simulink model "DTC_"  (R2023b)
settings: Solver=ode23tb  StartTime=0.0  StopTime=0.4  RelTol=1e-4
libraries: spsDCVoltageSourceLib x1, spsGroundLib x1, spsPermanentMagnetSynchronousMachineLib x1, spsThreePhaseVIMeasurementLib x1, spsUniversalBridgeLib x1, sps_lib x1
settings Model: Creator=rainy  LastModifiedBy=rainy
settings DebuggingCC: IgnoredZcDiagnostic=none

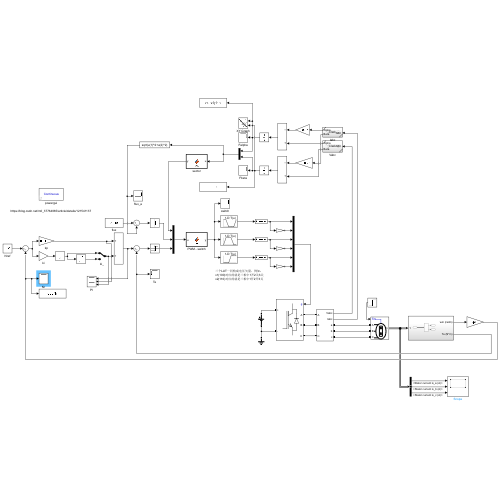
[thumbnail: Simulink's stored preview of the top-level diagram]
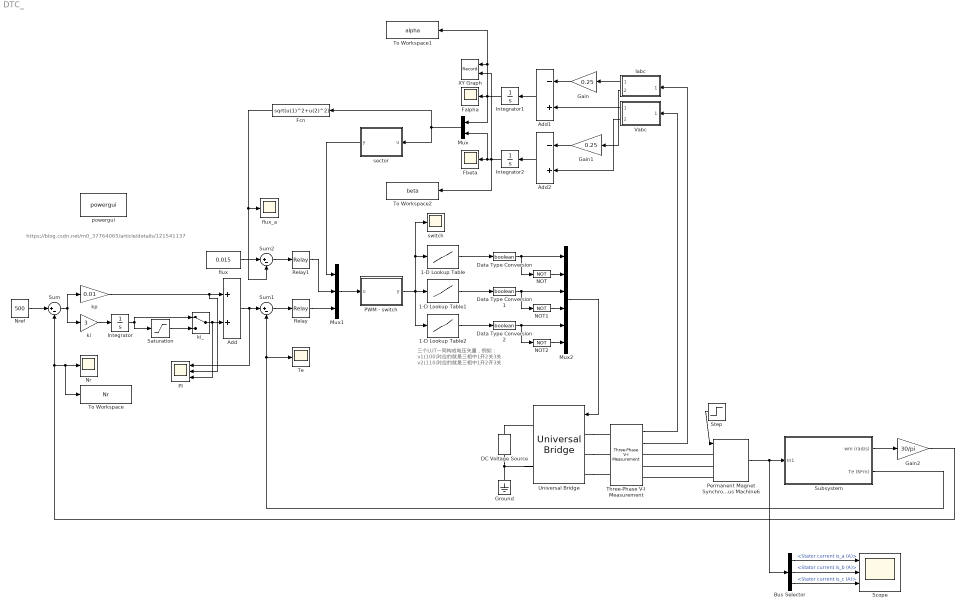
== system DTC_ ==
  note: 三个LUT一同构成电压矢量，例如：
      | v1(100)对应的就是三相中1开2关3关
      | v2(110)对应的就是三相中1开2开3关
  note: https://blog.csdn.net/m0_37764065/article/details/121541137
  1-D Lookup Table : Lookup_n-D  NumberOfTableDimensions=1  BreakpointsForDimension1=[1 2 3 4 5 6]  Table=[1 1 0 0 0 1]  InternalRulePriority=Speed  RndMeth=Simplest
  1-D Lookup Table1 : Lookup_n-D  NumberOfTableDimensions=1  BreakpointsForDimension1=[1 2 3 4 5 6]  Table=[0 1 1 1 0 0]  InternalRulePriority=Speed  RndMeth=Simplest
  1-D Lookup Table2 : Lookup_n-D  NumberOfTableDimensions=1  BreakpointsForDimension1=[1 2 3 4 5 6]  Table=[0 0 0 1 1 1]  InternalRulePriority=Speed  RndMeth=Simplest
  Add : Sum
  Add1 : Sum  Inputs=-+
  Add2 : Sum  Inputs=-+
  Bus Selector : BusSelector  OutputSignals=Stator current is_a (A),Stator current is_b (A),Stator current is_c (A)
  DC Voltage Source : spsDCVoltageSourceLib/DC Voltage Source  Amplitude=24  Measurements=Voltage
  Data Type Conversion : DataTypeConversion  OutDataTypeStr=boolean  SaturateOnIntegerOverflow=off  RndMeth=Floor
  Data Type Conversion1 : DataTypeConversion  OutDataTypeStr=boolean  SaturateOnIntegerOverflow=off  RndMeth=Floor
  Data Type Conversion2 : DataTypeConversion  OutDataTypeStr=boolean  SaturateOnIntegerOverflow=off  RndMeth=Floor
  Falpha : Scope
  Fbeta : Scope
  Fcn : Fcn  Expr=sqrt(u(1)^2+u(2)^2)
  Gain : Gain  Gain=0.25
  Gain1 : Gain  Gain=0.25
  Gain2 : Gain  Gain=30/pi
  Ground : spsGroundLib/Ground  LConnTagsString=a
  Iabc : Subsystem  ReferencedSubsystem=Clark
  Integrator : Integrator
  Integrator1 : Integrator
  Integrator2 : Integrator
  Mux : Mux  Inputs=2
  Mux1 : Mux  Inputs=3
  Mux2 : Mux  Inputs=6
  NOT : Logic  Operator=NOT  IconShape=distinctive  AllPortsSameDT=off  OutDataTypeStr=boolean
  NOT1 : Logic  Operator=NOT  IconShape=distinctive  AllPortsSameDT=off  OutDataTypeStr=boolean
  NOT2 : Logic  Operator=NOT  IconShape=distinctive  AllPortsSameDT=off  OutDataTypeStr=boolean
  Nr : Scope
  Nref : Constant  Value=500
  PI : Scope  NumInputPorts=3
  PWM - switch : MATLAB Function  TreatAsAtomicUnit=on
  Permanent Magnet Synchronous Machine6 : spsPermanentMagnetSynchronousMachineLib/Permanent Magnet Synchronous Machine  NbPhases=3  FluxDistribution=Sinusoidal  RotorType=Round  MechanicalLoad=Torque Tm  PresetModel=No  ShowDetailedParameters=on  MeasurementBus=off  Resistance=0.25  Inductance=8.5e-3  dqInductances=[8.5e-3,8.5e-3]  La=0.0005  MachineConstant=Flux linkage established by magnets (V.s)  Flux=0.01325  VoltageCst=9.6131  TorqueCst=0.0795  Flat=120  Mechanical=[0.00003 0 4 0]  PolePairs=4  InitialConditions=[0,0, 0,0]  InitialConditions5ph=[0 0 0 0 0 0]  RefAngle=Aligned with phase A axis (original Park)  IterativeDiscreteModel=Trapezoidal non iterative  TsBlock=-1  TsPowergui=0
  Relay : Relay  OnSwitchValue=0.01  OffSwitchValue=-0.01
  Relay1 : Relay  OnSwitchValue=0.002  OffSwitchValue=-0.002
  Saturation : Saturate  UpperLimit=10  LowerLimit=-10
  Scope : Scope  NumInputPorts=3
  Step : Step  Time=0.2  After=0.1  SampleTime=0
  Subsystem : Subsystem
  Sum : Sum  Inputs=|+-
  Sum1 : Sum  Inputs=|+-
  Sum2 : Sum  Inputs=|+-
  Te : Scope
  Three-Phase V-I Measurement : spsThreePhaseVIMeasurementLib/Three-Phase V-I Measurement  VoltageMeasurement=phase-to-ground  SetLabelV=off  LabelV=Vabc  Vpu=off  VpuLL=off  CurrentMeasurement=yes  SetLabelI=off  LabelI=Iabc  Ipu=off  Pbase=100e6  Vbase=500e3  OutputType=Complex  PhasorSimulation=off  PSBequivalent=0
  To Workspace : ToWorkspace  VariableName=Nr  SaveFormat=Timeseries  SampleTime=-1
  To Workspace1 : ToWorkspace  VariableName=alpha  SaveFormat=Timeseries  SampleTime=-1
  To Workspace2 : ToWorkspace  VariableName=beta  SaveFormat=Timeseries  SampleTime=-1
  Universal Bridge : spsUniversalBridgeLib/Universal Bridge  Arms=3  SnubberResistance=1e5  SnubberCapacitance=inf  Device=IGBT / Diodes  Ron=1e-3  Lon=0  ForwardVoltages="[  0  0  ]"  ForwardVoltage=0  GTOparameters=[ 10e-6 , 20e-6 ]  IGBTparameters=[ 1e-6 , 2e-6 ]  Measurements=None  Measurements_2=None  converterType=Rectifier
  Vabc : Subsystem  ReferencedSubsystem=Clark
  XY Graph : Record  FileSettingsInternal="{\"entries\":[{\"content\":{\"excelSettings\":{\"content\":{},\"type\":\"Streamout.ExcelSettings\"}},\"type\":\"Streamout.FileSettingStorage\",\"uuid\":\"\"}],\"packageUris\":[\"http:\\/\\/schema.mathworks.com\\/mf0\\/streamout_blocks\\/R2020a\"],\"version\":\"1.0\"}"  Layout=[1 1]  SignalsInternal="{\"entries\":[{\"content\":{\"signals\":[{\"content\":{\"blockPath\":[],\"dimensions\":[1],\"domain\":\"\",\"lineColor\":\"#22b573\",\"port\":1,\"sid\":[\"\"],\"signalID\":642,\"signalName\":\"Integrator1\"},\"type\":\"RecordBlkView.Signal\",\"uuid\":\"\"},{\"content\":{\"blockPath\":[],\"dimensions\":[1],\"domain\":\"\",\"lineColor\":\"#0072bd\",\"port\":2,\"sid\":[\"\"],\"signalID\":646,\"signalName\":\"Integrator2\"},\"type\":\"RecordBlkView.Signal\",\"uuid\":\"\"}]},\"type\":\"RecordBlkView.InputSignals\",\"uuid\":\"\"}],\"packageUris\":[\"http:\\/\\/schema.mathworks.com\\/mf0\\/streamout_blocks\\/R2020a\"],\"version\":\"1.0\"}"  VisualizationBindings="{\"xyplotplugin\":{\"info\":[{\"series\":[],\"subplotID\":1}]}}"  CompatibilityTag=XY  st=-1
  flux : Constant  Value=0.015
  flux_a : Scope
  ki : Gain  Gain=3
  ki_ : ManualSwitch
  kp : Gain  Gain=0.01
  powergui : sps_lib/powergui  Priority=1  SimulationMode=Continuous  SampleTime=50e-6  frequency=60  Iterations=50  frequencyindice=0  Pbase=100e6  ErrMax=1e-4  UnitsV=kV  UnitsW=MW  buscounter=0  FunctionMessages=off  echomessages=off  EnableUseOfTLC=off  CurrentSourceSwitches=off  DisableSnubberDevices=off  DisableRonSwitches=off  DisableVfSwitches=off  DisplayEquations=off  AutomaticDiscreteSolvers=off  SolverType=Tustin/Backward Euler (TBE)  Interpol=off  ExternalGateDelay=off  methode=off  Ts=100  x0status=blocks  SPID=on  SwTol=0  HookPort=off  NonlinearTolerance=1e-4  nMaxIteration=100  ContinueOnMaxIteration=off  RestoreLinks=warning  ResistiveCurrentMeasurement=off  Frange=[0:2:500]  Ylog=off  Xlog=on  ShowGrid=off  save=off  variable=ZData  structure=0  ZoomFFT=off  StartTime=0.0  cycles=1  DisplayStyle=1  fundamental=60  FreqAxis=off  MaxFrequency=1000  frequencyindicesteady=1  RmsSteady=1  display=off
  sector : MATLAB Function  TreatAsAtomicUnit=on
  switch : Scope
  wires:
  Sum/1 -> ki/1, kp/1
  ki/1 -> Integrator/1
  kp/1 -> PI/2, Add/1
  Add/1 -> PI/1, Sum1/1
  Gain2/1 -> Sum/2, To Workspace/1, Nr/1
  Nref/1 -> Sum/1
  Sum1/1 -> Relay/1
  Subsystem/2(Te (N*m)) -> Te/1, Sum1/2
  Subsystem/1(wm (rad/s)) -> Gain2/1
  flux/1 -> Sum2/1
  Sum2/1 -> Relay1/1
  Three-Phase V-I Measurement/1 -> Vabc/1
  Three-Phase V-I Measurement/2 -> Iabc/1
  Gain/1 -> Add1/1
  Iabc/1 -> Gain/1
  Vabc/1 -> Add1/2
  Add1/1 -> Integrator1/1
  Gain1/1 -> Add2/1
  Vabc/2 -> Add2/2
  Iabc/2 -> Gain1/1
  Add2/1 -> Integrator2/1
  Integrator1/1 -> To Workspace1/1, XY Graph/1, Mux/1, Falpha/1
  Integrator2/1 -> To Workspace2/1, XY Graph/2, Mux/2, Fbeta/1
  Mux/1 -> sector/1(u), Fcn/1
  Fcn/1 -> Sum2/2, flux_a/1
  Mux1/1 -> PWM - switch/1(u)
  Mux2/1 -> Universal Bridge/1
  Data Type Conversion/1 -> NOT/1, Mux2/1
  NOT/1 -> Mux2/2
  Data Type Conversion1/1 -> Mux2/3, NOT1/1
  NOT1/1 -> Mux2/4
  Data Type Conversion2/1 -> Mux2/5, NOT2/1
  NOT2/1 -> Mux2/6
  1-D Lookup Table/1 -> Data Type Conversion/1
  1-D Lookup Table1/1 -> Data Type Conversion1/1
  1-D Lookup Table2/1 -> Data Type Conversion2/1
  PWM - switch/1(y) -> 1-D Lookup Table2/1, switch/1, 1-D Lookup Table/1, 1-D Lookup Table1/1
  sector/1(y) -> Mux1/1
  Relay1/1 -> Mux1/2
  Relay/1 -> Mux1/3
  Integrator/1 -> ki_/1, Saturation/1
  ki_/1 -> PI/3, Add/2
  Saturation/1 -> ki_/2
  Bus Selector/1 -> Scope/1  "<Stator current is_a (A)>"
  Bus Selector/2 -> Scope/2  "<Stator current is_b (A)>"
  Bus Selector/3 -> Scope/3  "<Stator current is_c (A)>"
  Permanent Magnet Synchronous Machine6/1 -> Bus Selector/1, Subsystem/1(In1)
  Step/1 -> Permanent Magnet Synchronous Machine6/1
  connections:
  Universal Bridge/RConn2 -- DC Voltage Source/LConn1 -- Ground/LConn1
  DC Voltage Source/RConn1 -- Universal Bridge/RConn1
  Universal Bridge/LConn1 -- Three-Phase V-I Measurement/LConn1
  Universal Bridge/LConn2 -- Three-Phase V-I Measurement/LConn2
  Universal Bridge/LConn3 -- Three-Phase V-I Measurement/LConn3
  Permanent Magnet Synchronous Machine6/LConn1 -- Three-Phase V-I Measurement/RConn1
  Permanent Magnet Synchronous Machine6/LConn2 -- Three-Phase V-I Measurement/RConn2
  Permanent Magnet Synchronous Machine6/LConn3 -- Three-Phase V-I Measurement/RConn3

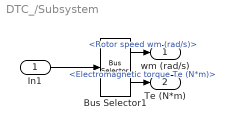
== system DTC_/Subsystem ==
  In1 : Inport
  Bus Selector1 : BusSelector  OutputSignals=Rotor speed wm (rad/s),Electromagnetic torque Te (N*m)
  wm (rad/s) : Outport
  Te (N*m) : Outport  Port=2
  wires:
  Bus Selector1/2 -> Te (N*m)/1  "<Electromagnetic torque Te (N*m)>"
  Bus Selector1/1 -> wm (rad/s)/1  "<Rotor speed wm (rad/s)>"
  In1/1 -> Bus Selector1/1

== matlab function DTC_/sector ==
  data: u input; y output
function y = fcn(u)

if(u(2) == 0)
    N = 3;
else
    % 将\psi_{\aplha}和\psi_{\beta}分解为三相
    a1 = u(1);
    b1 = u(1)*(-0.5) + sqrt(3)/2*u(2);
    c1 = u(1)*(-0.5) - sqrt(3)/2*u(2);
    
    % a1 > 0，有扇区126
    % b1 > 0，有扇区234
    % c1 > 0，有扇区456
    % n为a1 b1 c1中>0的个数，0 < n < 3
    % 
    % a b c | s
    %-------|---
    % 0 0 1 | 2
    % 0 1 0 | 6
    % 0 1 1 | 1
    % 1 0 0 | 4
    % 1 0 1 | 3
    % 1 1 0 | 5

    if(a1 > 0)
        a = 0;
    else
        a = 1;
    end
    
    if(b1 > 0)
        b = 0;
    else
        b = 1;
    end
    
    if(c1 > 0)
        c = 0;
    else
        c = 1;
    end

    N = 4*a+2*b+c;
end

Sector_table=[2 6 1 4 3 5];

y = Sector_table(N);

== matlab function DTC_/PWM - switch ==
  data: u input; y output
function y = fcn(u)

% u(1) 扇区
% u(2) 磁链
% u(3) 转矩

V_Table=[5 6 1 2 3 4;3 4 5 6 1 2;6 1 2 3 4 5;2 3 4 5 6 1];
x=2*u(2)+u(3)+1;

y = V_Table(x, u(1));
